simulink model "e4"  (R2024b)
settings: Solver=VariableStepAuto  StartTime=0.0  StopTime=10.0  RelTol=1e-3
settings Model: Creator=Lenovo  LastModifiedBy=Lenovo

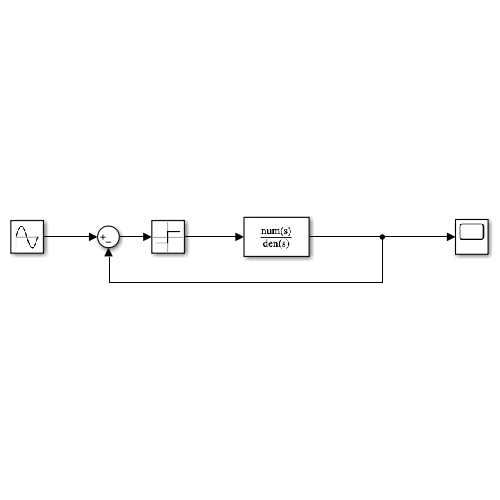
[thumbnail: Simulink's stored preview of the top-level diagram]
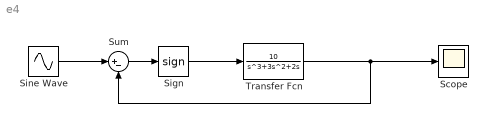
== system e4 ==
  Scope : Scope
  Sign : Signum
  Sine Wave : Sin  SampleTime=0
  Sum : Sum  Inputs=|+-
  Transfer Fcn : TransferFcn  Numerator=[0 10]  Denominator=[1 3 2 0]
  wires:
  Sign/1 -> Transfer Fcn/1
  Sum/1 -> Sign/1
  Sine Wave/1 -> Sum/1
  Transfer Fcn/1 -> Sum/2, Scope/1
